simulink model "dynamics"  (R2017b)
settings: Solver=VariableStepAuto  StartTime=0.0  StopTime=10.0  RelTol=1e-3
undefined symbols (not defined in the file or in its folder): AU, c, Cube, G, mu_s, SC, Sun, Switch
settings Model: Creator=shriyahazra  LastModifiedBy=hazr_sh

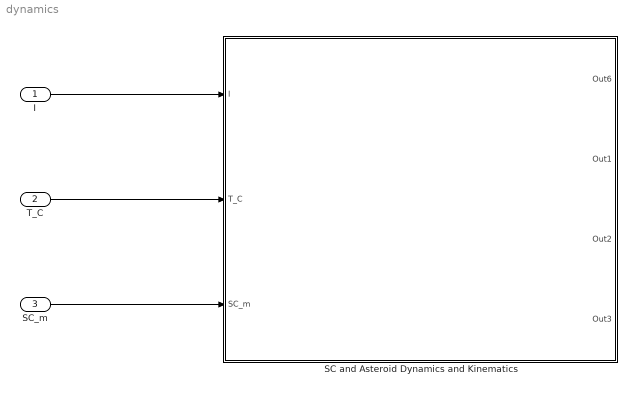
== system dynamics ==
  I : Inport
  T_C : Inport  Port=2
  SC_m : Inport  Port=3
  SC and Asteroid Dynamics and Kinematics : Subsystem
  wires:
  I/1 -> SC and Asteroid Dynamics and Kinematics/1(I)
  T_C/1 -> SC and Asteroid Dynamics and Kinematics/2(T_C)
  SC_m/1 -> SC and Asteroid Dynamics and Kinematics/3(SC_m)

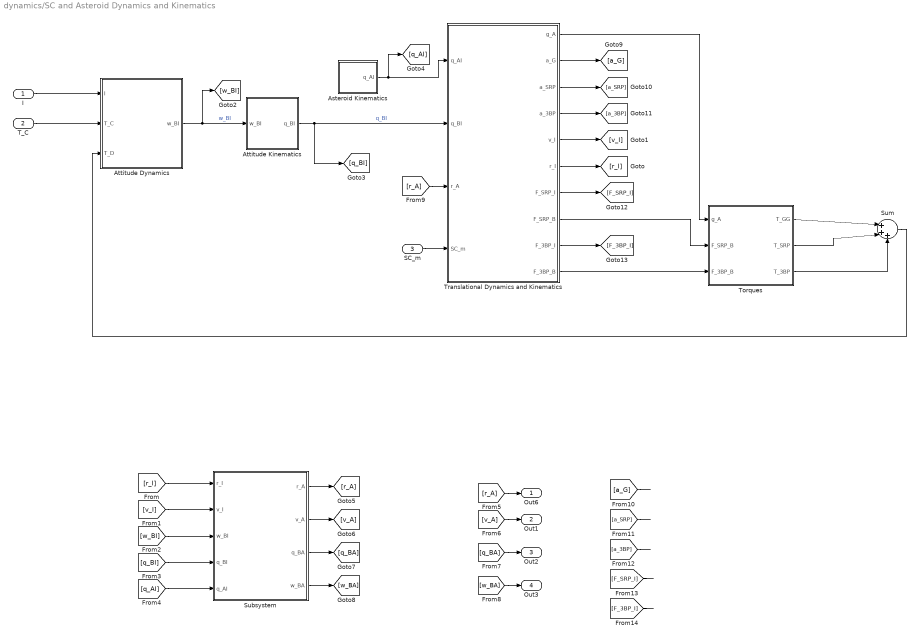
== system dynamics/SC and Asteroid Dynamics and Kinematics ==
  I : Inport
  T_C : Inport  Port=2
  SC_m : Inport  Port=3
  Asteroid Kinematics : Subsystem
  Attitude Dynamics : Subsystem
  Attitude Kinematics : Subsystem
  Subsystem : Subsystem
  Sum : Sum  Inputs=|+++
  Torques : Subsystem
  Translational Dynamics and Kinematics : Subsystem
  Out6 : Outport
  Out1 : Outport  Port=2
  Out2 : Outport  Port=3
  Out3 : Outport  Port=4
  wires:
  SC_m/1 -> Translational Dynamics and Kinematics/4(SC_m)
  [a_G] -> ?
  [a_3BP] -> ?
  [v_A] -> Out1/1
  [q_BA] -> Out2/1
  [w_BA] -> Out3/1
  [a_SRP] -> ?
  Translational Dynamics and Kinematics/1(g_A) -> Torques/1(g_A)
  [r_A] -> Out6/1
  T_C/1 -> Attitude Dynamics/2(T_C)
  Attitude Kinematics/1(q_BI) -> [q_BI], Translational Dynamics and Kinematics/2(q_BI)  "q_BI"
  [r_I] -> Subsystem/1(r_I)
  [r_A] -> Translational Dynamics and Kinematics/3(r_A)
  Translational Dynamics and Kinematics/5(v_I) -> [v_I]
  Translational Dynamics and Kinematics/6(r_I) -> [r_I]
  [q_AI] -> Subsystem/5(q_AI)
  Torques/2(T_SRP) -> Sum/2
  Asteroid Kinematics/1(q_AI) -> Translational Dynamics and Kinematics/1(q_AI), [q_AI]
  Translational Dynamics and Kinematics/4(a_3BP) -> [a_3BP]
  I/1 -> Attitude Dynamics/1(I)
  Attitude Dynamics/1(w_BI) -> [w_BI], Attitude Kinematics/1(w_BI)  "w_BI"
  Subsystem/3(q_BA) -> [q_BA]
  Translational Dynamics and Kinematics/3(a_SRP) -> [a_SRP]
  Torques/3(T_3BP) -> Sum/3
  Translational Dynamics and Kinematics/2(a_G) -> [a_G]
  [w_BI] -> Subsystem/3(w_BI)
  Sum/1 -> Attitude Dynamics/3(T_D)
  Torques/1(T_GG) -> Sum/1
  Subsystem/2(v_A) -> [v_A]
  [v_I] -> Subsystem/2(v_I)
  [q_BI] -> Subsystem/4(q_BI)
  Subsystem/4(w_BA) -> [w_BA]
  Subsystem/1(r_A) -> [r_A]
  Translational Dynamics and Kinematics/8(F_SRP_B) -> Torques/2(F_SRP_B)
  Translational Dynamics and Kinematics/10(F_3BP_B) -> Torques/3(F_3BP_B)
  Translational Dynamics and Kinematics/7(F_SRP_I) -> [F_SRP_I]
  Translational Dynamics and Kinematics/9(F_3BP_I) -> [F_3BP_I]
  [F_SRP_I] -> ?
  [F_3BP_I] -> ?

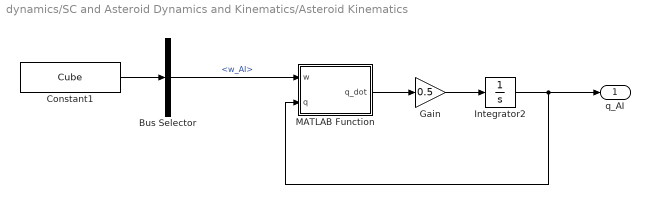
== system dynamics/SC and Asteroid Dynamics and Kinematics/Asteroid Kinematics ==
  Bus Selector : BusSelector  OutputSignals=w_AI
  Constant1 : Constant  Value=Cube  VectorParams1D=off  OutDataTypeStr=Bus: slBus1
  Gain : Gain  Gain=0.5
  Integrator2 : Integrator  InitialCondition=[0 0 0 0]'
  MATLAB Function : MATLAB Function  TreatAsAtomicUnit=on
  q_AI : Outport
  wires:
  MATLAB Function/1(q_dot) -> Gain/1
  Gain/1 -> Integrator2/1
  Bus Selector/1 -> MATLAB Function/1(w)  "<w_AI>"
  Integrator2/1 -> MATLAB Function/2(q), q_AI/1
  Constant1/1 -> Bus Selector/1

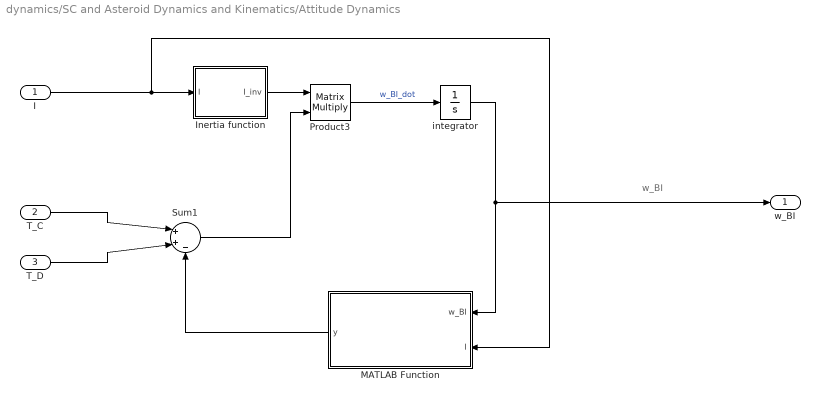
== system dynamics/SC and Asteroid Dynamics and Kinematics/Attitude Dynamics ==
  note: w_BI
  I : Inport
  T_C : Inport  Port=2
  T_D : Inport  Port=3
  " integrator" : Integrator  InitialCondition=[0,0,0]'
  "Inertia function " : MATLAB Function  TreatAsAtomicUnit=on
  MATLAB Function : MATLAB Function  TreatAsAtomicUnit=on
  Product3 : Product  Multiplication=Matrix(*)
  Sum1 : Sum  Inputs=|++-
  w_BI : Outport
  wires:
  " integrator"/1 -> w_BI/1, MATLAB Function/1(w_BI)
  I/1 -> MATLAB Function/2(I), "Inertia function "/1(I)
  T_C/1 -> Sum1/1
  "Inertia function "/1(I_inv) -> Product3/1
  MATLAB Function/1(y) -> Sum1/3
  Sum1/1 -> Product3/2
  Product3/1 -> " integrator"/1  "w_BI_dot"
  T_D/1 -> Sum1/2

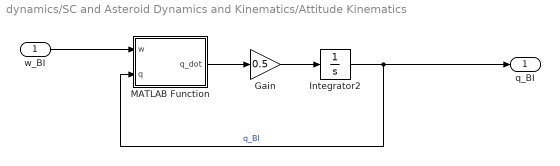
== system dynamics/SC and Asteroid Dynamics and Kinematics/Attitude Kinematics ==
  w_BI : Inport
  Gain : Gain  Gain=0.5
  Integrator2 : Integrator  InitialCondition=[0 0 0 0]'
  MATLAB Function : MATLAB Function  TreatAsAtomicUnit=on
  q_BI : Outport
  wires:
  w_BI/1 -> MATLAB Function/1(w)
  Integrator2/1 -> MATLAB Function/2(q), q_BI/1  "q_BI"
  MATLAB Function/1(q_dot) -> Gain/1
  Gain/1 -> Integrator2/1

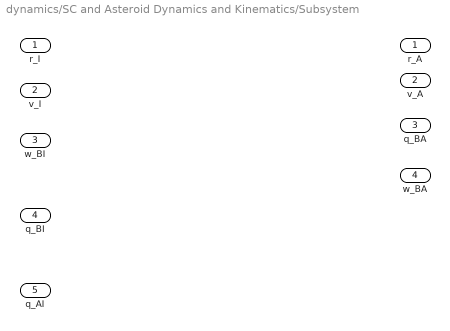
== system dynamics/SC and Asteroid Dynamics and Kinematics/Subsystem ==
  r_I : Inport
  v_I : Inport  Port=2
  w_BI : Inport  Port=3
  q_BI : Inport  Port=4
  q_AI : Inport  Port=5
  r_A : Outport
  v_A : Outport  Port=2
  q_BA : Outport  Port=3
  w_BA : Outport  Port=4

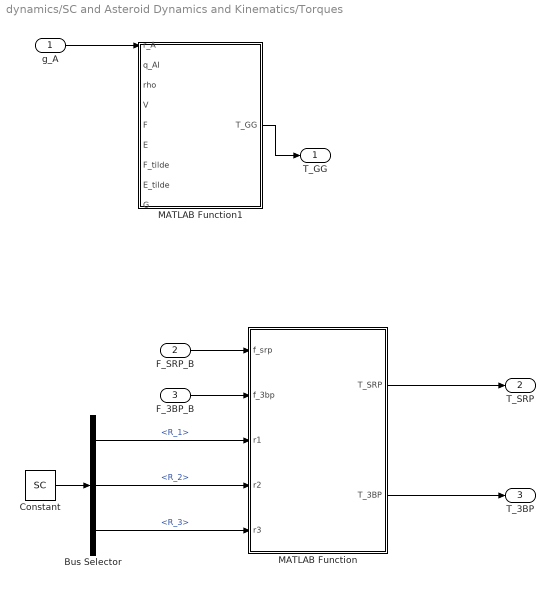
== system dynamics/SC and Asteroid Dynamics and Kinematics/Torques ==
  g_A : Inport
  F_SRP_B : Inport  Port=2
  F_3BP_B : Inport  Port=3
  Bus Selector : BusSelector  OutputSignals=Polyhedron.R_1,Polyhedron.R_2,Polyhedron.R_3
  Constant : Constant  Value=SC  OutDataTypeStr=Bus: slBus3
  MATLAB Function : MATLAB Function  TreatAsAtomicUnit=on
  MATLAB Function1 : MATLAB Function  TreatAsAtomicUnit=on
  T_GG : Outport
  T_SRP : Outport  Port=2
  T_3BP : Outport  Port=3
  wires:
  g_A/1 -> MATLAB Function1/1(r_A)
  F_SRP_B/1 -> MATLAB Function/1(f_srp)
  Constant/1 -> Bus Selector/1
  Bus Selector/1 -> MATLAB Function/3(r1)  "<R_1>"
  Bus Selector/2 -> MATLAB Function/4(r2)  "<R_2>"
  MATLAB Function/1(T_SRP) -> T_SRP/1
  F_3BP_B/1 -> MATLAB Function/2(f_3bp)
  MATLAB Function/2(T_3BP) -> T_3BP/1
  MATLAB Function1/1(T_GG) -> T_GG/1
  Bus Selector/3 -> MATLAB Function/5(r3)  "<R_3>"

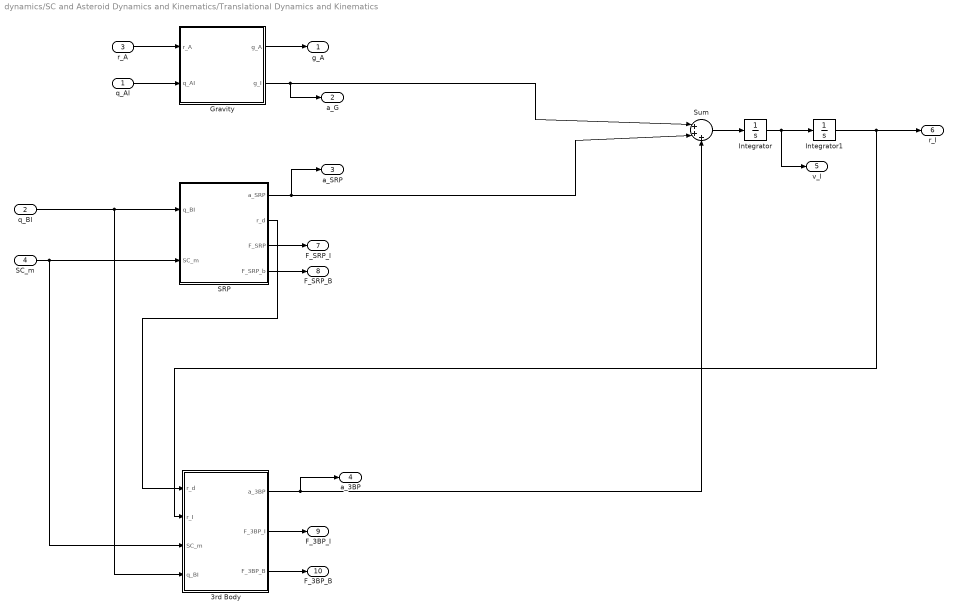
== system dynamics/SC and Asteroid Dynamics and Kinematics/Translational Dynamics and Kinematics ==
  q_AI : Inport
  q_BI : Inport  Port=2
  r_A : Inport  Port=3
  SC_m : Inport  Port=4
  3rd Body : Subsystem
  Gravity : Subsystem
  Integrator : Integrator  InitialCondition=SC.vinit
  Integrator1 : Integrator  InitialCondition=SC.xinit
  SRP : Subsystem
  Sum : Sum  Inputs=|+++
  g_A : Outport
  a_G : Outport  Port=2
  a_SRP : Outport  Port=3
  a_3BP : Outport  Port=4
  v_I : Outport  Port=5
  r_I : Outport  Port=6
  F_SRP_I : Outport  Port=7
  F_SRP_B : Outport  Port=8
  F_3BP_I : Outport  Port=9
  F_3BP_B : Outport  Port=10
  wires:
  SRP/1(a_SRP) -> Sum/2, a_SRP/1
  SRP/2(r_d) -> 3rd Body/1(r_d)
  3rd Body/1(a_3BP) -> a_3BP/1, Sum/3
  Sum/1 -> Integrator/1
  Integrator/1 -> v_I/1, Integrator1/1
  Gravity/2(g_I) -> a_G/1, Sum/1
  q_BI/1 -> SRP/1(q_BI), 3rd Body/4(q_BI)
  Gravity/1(g_A) -> g_A/1
  Integrator1/1 -> 3rd Body/2(r_I), r_I/1
  r_A/1 -> Gravity/1(r_A)
  q_AI/1 -> Gravity/2(q_AI)
  SRP/3(F_SRP) -> F_SRP_I/1
  3rd Body/2(F_3BP_I) -> F_3BP_I/1
  SC_m/1 -> 3rd Body/3(SC_m), SRP/2(SC_m)
  SRP/4(F_SRP_b) -> F_SRP_B/1
  3rd Body/3(F_3BP_B) -> F_3BP_B/1

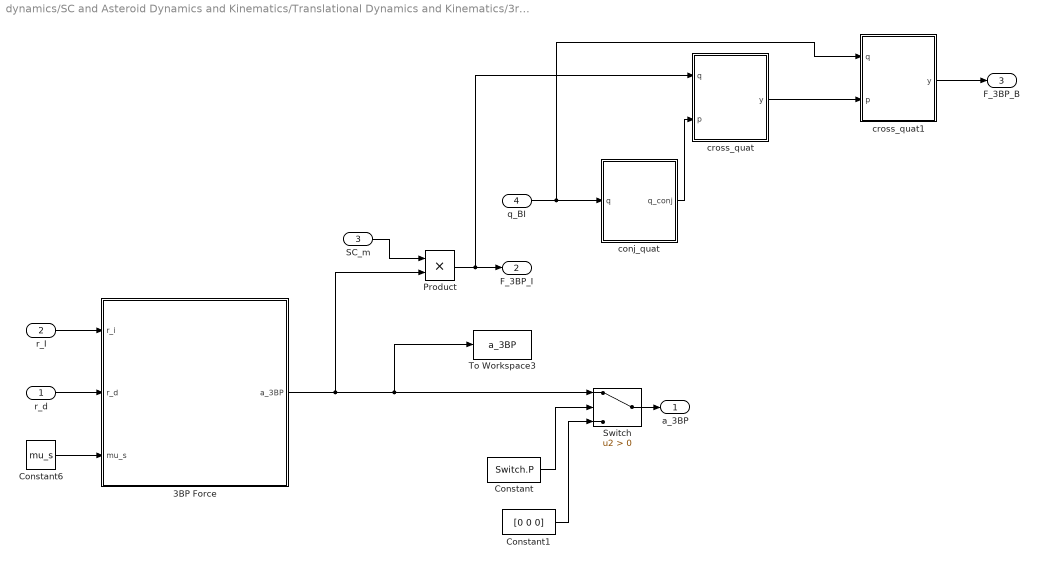
== system dynamics/SC and Asteroid Dynamics and Kinematics/Translational Dynamics and Kinematics/3rd Body ==
  r_d : Inport
  r_I : Inport  Port=2
  SC_m : Inport  Port=3
  q_BI : Inport  Port=4
  3BP Force : MATLAB Function  TreatAsAtomicUnit=on
  Constant : Constant  Value=Switch.P
  Constant1 : Constant  Value=[0 0 0]
  Constant6 : Constant  Value=mu_s
  Product : Product
  Switch : Switch  Criteria=u2 > Threshold
  To Workspace3 : ToWorkspace  VariableName=a_3BP  SampleTime=-1
      settings: Save2DSignal=2-D array (concatenate along first dimension)
  conj_quat : MATLAB Function  TreatAsAtomicUnit=on
  cross_quat : MATLAB Function  TreatAsAtomicUnit=on
  cross_quat1 : MATLAB Function  TreatAsAtomicUnit=on
  a_3BP : Outport
  F_3BP_I : Outport  Port=2
  F_3BP_B : Outport  Port=3
  wires:
  Constant6/1 -> 3BP Force/3(mu_s)
  r_I/1 -> 3BP Force/1(r_i)
  r_d/1 -> 3BP Force/2(r_d)
  3BP Force/1(a_3BP) -> Product/2, To Workspace3/1, Switch/1
  Switch/1 -> a_3BP/1
  Constant/1 -> Switch/2
  Constant1/1 -> Switch/3
  Product/1 -> cross_quat/1(q), F_3BP_I/1
  SC_m/1 -> Product/1
  cross_quat/1(y) -> cross_quat1/2(p)
  conj_quat/1(q_conj) -> cross_quat/2(p)
  q_BI/1 -> conj_quat/1(q), cross_quat1/1(q)
  cross_quat1/1(y) -> F_3BP_B/1

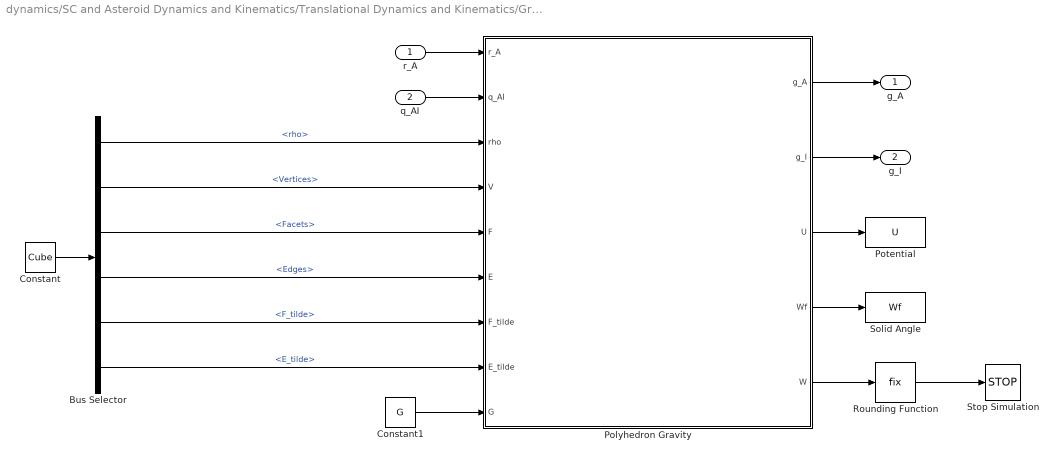
== system dynamics/SC and Asteroid Dynamics and Kinematics/Translational Dynamics and Kinematics/Gravity ==
  r_A : Inport
  q_AI : Inport  Port=2
  Bus Selector : BusSelector  OutputSignals=rho,Polyhedron.Vertices,Polyhedron.Facets,Polyhedron.Edges,Polyhedron.F_tilde,Polyhedron.E_tilde
  Constant : Constant  Value=Cube  VectorParams1D=off  OutDataTypeStr=Bus: slBus1
  Constant1 : Constant  Value=G
  Polyhedron Gravity : MATLAB Function  TreatAsAtomicUnit=on
  Potential : ToWorkspace  VariableName=U  SaveFormat=Timeseries  SampleTime=-1
  Rounding Function : Rounding  Operator=fix
  Solid Angle : ToWorkspace  VariableName=Wf  SaveFormat=Timeseries  SampleTime=-1
  Stop Simulation : Stop
  g_A : Outport
  g_I : Outport  Port=2
  wires:
  Bus Selector/5 -> Polyhedron Gravity/7(F_tilde)  "<F_tilde>"
  Polyhedron Gravity/4(Wf) -> Solid Angle/1
  Constant1/1 -> Polyhedron Gravity/9(G)
  Bus Selector/6 -> Polyhedron Gravity/8(E_tilde)  "<E_tilde>"
  Constant/1 -> Bus Selector/1
  Bus Selector/4 -> Polyhedron Gravity/6(E)  "<Edges>"
  Bus Selector/1 -> Polyhedron Gravity/3(rho)  "<rho>"
  Bus Selector/2 -> Polyhedron Gravity/4(V)  "<Vertices>"
  Bus Selector/3 -> Polyhedron Gravity/5(F)  "<Facets>"
  Polyhedron Gravity/3(U) -> Potential/1
  Polyhedron Gravity/1(g_A) -> g_A/1
  r_A/1 -> Polyhedron Gravity/1(r_A)
  q_AI/1 -> Polyhedron Gravity/2(q_AI)
  Polyhedron Gravity/2(g_I) -> g_I/1
  Polyhedron Gravity/5(W) -> Rounding Function/1
  Rounding Function/1 -> Stop Simulation/1

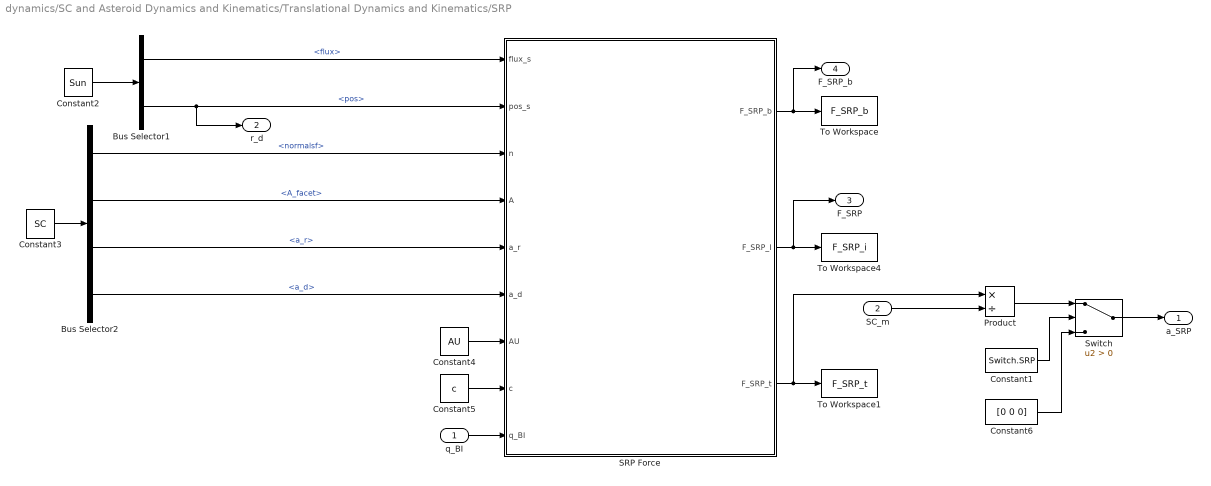
== system dynamics/SC and Asteroid Dynamics and Kinematics/Translational Dynamics and Kinematics/SRP ==
  q_BI : Inport
  SC_m : Inport  Port=2
  Bus Selector1 : BusSelector  OutputSignals=flux,pos
  Bus Selector2 : BusSelector  OutputSignals=Polyhedron.normalsf,Polyhedron.A_facet,a_r,a_d
  Constant1 : Constant  Value=Switch.SRP
  Constant2 : Constant  Value=Sun  VectorParams1D=off  OutDataTypeStr=Bus: slBus2
  Constant3 : Constant  Value=SC  VectorParams1D=off  OutDataTypeStr=Bus: slBus3
  Constant4 : Constant  Value=AU
  Constant5 : Constant  Value=c
  Constant6 : Constant  Value=[0 0 0]
  Product : Product  Inputs=*/
  SRP Force : MATLAB Function  TreatAsAtomicUnit=on
  Switch : Switch  Criteria=u2 > Threshold
  To Workspace : ToWorkspace  VariableName=F_SRP_b  SampleTime=-1
      settings: Save2DSignal=2-D array (concatenate along first dimension)
  To Workspace1 : ToWorkspace  VariableName=F_SRP_t  SampleTime=-1
      settings: Save2DSignal=2-D array (concatenate along first dimension)
  To Workspace4 : ToWorkspace  VariableName=F_SRP_i  SampleTime=-1
      settings: Save2DSignal=2-D array (concatenate along first dimension)
  a_SRP : Outport
  r_d : Outport  Port=2
  F_SRP : Outport  Port=3
  F_SRP_b : Outport  Port=4
  wires:
  Bus Selector2/2 -> SRP Force/4(A)  "<A_facet>"
  Bus Selector2/4 -> SRP Force/6(a_d)  "<a_d>"
  Bus Selector1/2 -> r_d/1, SRP Force/2(pos_s)  "<pos>"
  Constant3/1 -> Bus Selector2/1
  Constant2/1 -> Bus Selector1/1
  Bus Selector2/1 -> SRP Force/3(n)  "<normalsf>"
  Bus Selector2/3 -> SRP Force/5(a_r)  "<a_r>"
  Constant4/1 -> SRP Force/7(AU)
  q_BI/1 -> SRP Force/9(q_BI)
  Constant5/1 -> SRP Force/8(c)
  SRP Force/1(F_SRP_b) -> F_SRP_b/1, To Workspace/1
  SRP Force/2(F_SRP_I) -> F_SRP/1, To Workspace4/1
  SRP Force/3(F_SRP_t) -> To Workspace1/1, Product/1
  Bus Selector1/1 -> SRP Force/1(flux_s)  "<flux>"
  SC_m/1 -> Product/2
  Product/1 -> Switch/1
  Constant1/1 -> Switch/2
  Switch/1 -> a_SRP/1
  Constant6/1 -> Switch/3

== matlab function dynamics/SC and Asteroid Dynamics and Kinematics/Translational Dynamics and Kinematics/SRP/SRP Force ==
  data: flux_s input; pos_s input; n input; A input; a_r input; a_d input; AU input; c input; F_SRP_b output; F_SRP_I output; F_SRP_t output; q_BI input
function [F_SRP_b,F_SRP_I,F_SRP_t]   = F_SRP(flux_s,pos_s,n,A,a_r,a_d,AU,c,q_BI)
%% This function generates SRP force per facet in the body and inertial frame of reference
%Inputs:
%flux_s, pos_s = Sun flux and position 
%n = facet normals, 
%A = facet area, 
%a_r,a_d = specular and diffuse reflectivity

e = pos_s(1,1:3)/norm(pos_s(1,1:3));  %presently just postion vector of sun from asteroid in the inertial frame of reference can be resolved per facet 
P = flux_s/((pos_s(1,1:3)/AU)^2*c);   %radiation pressure at the distance of the asteroid

F_SRP_b = zeros(size(n,1),3); 
for i=1:1:size(n,1)
    
    co = dot(n(i,1:3),e(1,1:3),2);

    if i<=12 %change as per number of normals representing the main body and solar arrays of SC
        F = -P*A(i,:)*co.*((2*(a_d(1,1)/3 + a_r(1,1)*co))'.*n(i,1:3) + (1-a_r(1,1))'.*e);
        F_SRP_b(i,:) = F;
    else
        F = -P*A(i,:)*co.*((2*(a_d(1,2)/3 + a_r(1,2)*co))'.*n(i,1:3) + (1-a_r(1,2))'.*e);
        F_SRP_b(i,:) = F;
    end
    
    
end
% 
F_SRP_I = cross_quat(q_BI,cross_quat([F_SRP_b 0]',conj_quat(q_BI)));
F_SRP_t = sum(F_SRP_b);

end

== matlab function dynamics/SC and Asteroid Dynamics and Kinematics/Translational Dynamics and Kinematics/Gravity/Polyhedron Gravity ==
  data: r_A input; q_AI input; rho input; V input; F input; E input; F_tilde input; E_tilde input; g_A output; g_I output; G input; U output; Wf output; W output
function [g_A,g_I, U, Wf,W] = Poly_gravity(r_A,q_AI,rho,V,F,E,F_tilde,E_tilde,G)
%% Function to calculate Cube gravity from Asteroid structure (from Get_Asteroid function)
%
% Inputs: r_A - position of a field point in Asteroid frame
%         Asteroid - Asteroid structure
%
% Outputs: g_A - gravitational acceleration in Asteroid frame
%          U - gravitational potential in Asteroid frame
%          Wf - THE solid angle, which shows whether the point is in or out
%               It can be used for stopping simulation if SC crashes

%% Initialization

Wf = 0;

Facets = [0 0 0]';
Edges = [0 0 0]';

U_edg = 0;
U_fac = 0;

S = r_A;

for j=1:1:size(E,1)
    
    % Calculate gravity due to edge potential
    
    R1 = V(E(j,1),:);    
    R2 = V(E(j,2),:);    

    Ri = R1'-S;
    ri = norm(Ri);
    
    Rj = R2'-S;
    rj = norm(Rj);
        
    Rij = Rj-Ri;
    eij = norm(Rij);

    Re1 =(Ri+Rj)/2;
   
    Le = log((ri+rj+eij)/(ri+rj-eij));
    
    if Le == Inf
     
        Le = 0;
     
    end
    
    Edges = (Le*E_tilde(:,:,j)*Re1)+Edges;
    U_edg = (Le*Re1'*E_tilde(:,:,j)*Re1)+U_edg;
    
end

 for i=1:1:(size(F,1))
    
    % Calculate gravity due to face potential
    
    R1 = V(F(i,1),:);    
    R2 = V(F(i,2),:);    
    R3 = V(F(i,3),:);
    

    Ri = R1'-S;
    ri = norm(Ri);
    
    Rj = R2'-S;
    rj = norm(Rj);
    
    Rk = R3'-S;
    rk = norm(Rk);
    
    
    wf = 2*atan2(dot(Ri, cross(Rj,Rk)),(ri*rj*rk+ri*dot(Rj,Rk)+rj*dot(Rk,Ri)+rk*dot(Ri,Rj)));
    
    Rf =(Ri+Rj+Rk)/3;

    U_fac = wf*Rf'*F_tilde(:,:,i)*Rf+U_fac;
    Facets = wf*F_tilde(:,:,i)*Rf+Facets;
    
    Wf = wf+Wf;
  
 end

g_A = G*rho*(-Edges+Facets);
g_I = cross_quat(conj_quat(q_AI),cross_quat(g_A,q_AI));

U = 0.5*G*rho*(U_edg-U_fac);

if Wf>10
    W=1;
else
    W=0;
end
end

== matlab function dynamics/SC and Asteroid Dynamics and Kinematics/Translational Dynamics and Kinematics/3rd Body/3BP Force ==
  data: r_i input; a_3BP output; r_d input; mu_s input
function a_3BP   = F_3BP(r_i,r_d,mu_s)

r_id = r_d - r_i;
a_3BP = -mu_s*(r_id/norm(r_id)^3 - r_d/norm(r_d)^3); 

end

== matlab function dynamics/SC and Asteroid Dynamics and Kinematics/Asteroid Kinematics/MATLAB Function ==
  data: w input; q_dot output; q input
function q_dot = fcn(w,q)

W = [0     w(3) -w(2) w(1)
    -w(3)  0     w(1) w(2)
     w(2) -w(1)  0    w(3)
    -w(1) -w(2) -w(3) 0];

q_dot = W*q;

end

== matlab function dynamics/SC and Asteroid Dynamics and Kinematics/Attitude Dynamics/MATLAB Function ==
  data: w_BI input; I input; y output
function y = fcn(w_BI,I)

y = cross(w_BI, I*w_BI);

end

== matlab function dynamics/SC and Asteroid Dynamics and Kinematics/Attitude Kinematics/MATLAB Function ==
  data: w input; q_dot output; q input
function q_dot = fcn(w,q)

W = [0 w(3) -w(2) w(1)
         -w(3) 0 w(1) w(2)
         w(2) -w(1) 0 w(3)
         -w(1) -w(2) -w(3) 0];

q_dot = w*q;

end

== matlab function dynamics/SC and Asteroid Dynamics and Kinematics/Attitude Dynamics/Inertia function  ==
  data: I_inv output; I input
function I_inv = fcn(I)

I_inv = inv(I);

end

== matlab function dynamics/SC and Asteroid Dynamics and Kinematics/Torques/MATLAB Function ==
  data: f_srp input; f_3bp input; T_SRP output; r1 input; r2 input; r3 input; T_3BP output
function [T_SRP,T_3BP] = Torques(f_srp,f_3bp,r1,r2,r3)

c = (r1+r2+r3)/3;
t = zeros(size(f_srp));

for i = 1:length(f_srp)
    t(i,:) = cross(c(i,:),f_srp(i,:));
    t2(i,:) = cross(c(i,:),f_3bp);
end

    T_SRP = sum(t);
    T_3BP = sum(t2);
end

== matlab function dynamics/SC and Asteroid Dynamics and Kinematics/Translational Dynamics and Kinematics/3rd Body/cross_quat ==
  data: q input; y output; p input
function y = cross_quat(q, p)
% Quaternion Cross Product

q4= q(4);
p4= p(4);

q_vect= q(1:3);
p_vect= p(1:3);

y = [q4.*p_vect + p4.*q_vect - cross(q_vect, p_vect); q4*p4 - dot(q_vect,p_vect)];
end

== matlab function dynamics/SC and Asteroid Dynamics and Kinematics/Translational Dynamics and Kinematics/3rd Body/conj_quat ==
  data: q input; q_conj output
function q_conj = conj_quat(q)
%Unit quaternion conjugation

q0= q(4);
q_vect= q(1:3);

q_conj = [-q_vect; q0];
end

== matlab function dynamics/SC and Asteroid Dynamics and Kinematics/Translational Dynamics and Kinematics/3rd Body/cross_quat1 ==
  data: q input; y output; p input
function y = cross_quat(q, p)
% Quaternion Cross Product

q4= q(4);
p4= p(4);

q_vect= q(1:3);
p_vect= p(1:3);

y = [q4.*p_vect + p4.*q_vect - cross(q_vect, p_vect); q4*p4 - dot(q_vect,p_vect)];
end

== matlab function dynamics/SC and Asteroid Dynamics and Kinematics/Torques/MATLAB Function1 ==
  data: r_A input; T_GG output; q_AI input; rho input; V input; F input; E input; F_tilde input; E_tilde input; G input
function T_GG = Torque_GG(r_A,q_AI,rho,V,F,E,F_tilde,E_tilde,G)


 [g_A,g_I, U, Wf,W] = Poly_gravity(r_A,q_AI,rho,V,F,E,F_tilde,E_tilde,G)

 
 
 
 T_GG =;

end
